simulink model "simulacionPID"  (R2020a)
settings: Solver=VariableStepAuto  StartTime=0.0  StopTime=10.0  RelTol=1e-3
undefined symbols (not defined in the file): x, xg, y, yg
settings Model: Creator=nacho  LastModifiedBy=nacho

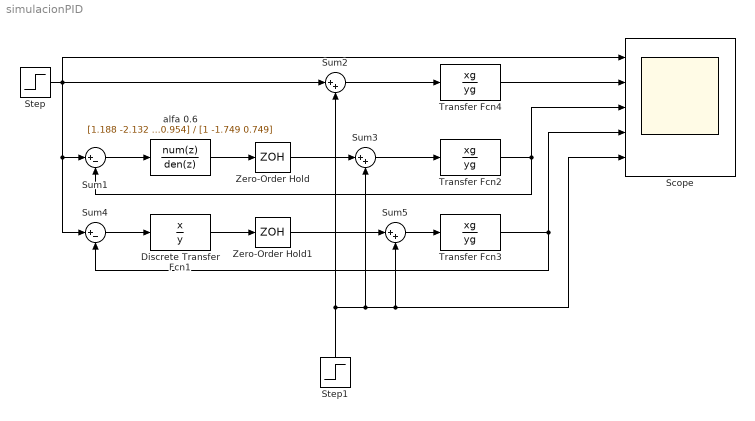
== system simulacionPID ==
  Discrete Transfer Fcn1 : DiscreteTransferFcn  Numerator=x  Denominator=y  SampleTime=0.03
  Scope : Scope  NumInputPorts=5
  Step : Step  Time=0.5  SampleTime=0.001
  Step1 : Step  Time=5  SampleTime=0.001
  Sum1 : Sum  Inputs=|+-
  Sum2 : Sum  Inputs=|++
  Sum3 : Sum  Inputs=|++
  Sum4 : Sum  Inputs=|+-
  Sum5 : Sum  Inputs=|++
  Transfer Fcn2 : TransferFcn  Numerator=xg  Denominator=yg
  Transfer Fcn3 : TransferFcn  Numerator=xg  Denominator=yg
  Transfer Fcn4 : TransferFcn  Numerator=xg  Denominator=yg
  Zero-Order Hold : ZeroOrderHold  SampleTime=0.03
  Zero-Order Hold1 : ZeroOrderHold  SampleTime=0.03
  alfa 0.6 : DiscreteTransferFcn  Numerator=[1.188 -2.132 0.954]  Denominator=[1 -1.749 0.749]  SampleTime=0.03
  wires:
  Transfer Fcn4/1 -> Scope/2
  Transfer Fcn2/1 -> Scope/3, Sum1/2
  alfa 0.6/1 -> Zero-Order Hold/1
  Sum1/1 -> alfa 0.6/1
  Sum2/1 -> Transfer Fcn4/1
  Zero-Order Hold/1 -> Sum3/1
  Sum3/1 -> Transfer Fcn2/1
  Discrete Transfer Fcn1/1 -> Zero-Order Hold1/1
  Step1/1 -> Scope/5, Sum5/2, Sum3/2, Sum2/2
  Transfer Fcn3/1 -> Scope/4, Sum4/2
  Step/1 -> Sum2/1, Scope/1, Sum4/1, Sum1/1
  Sum4/1 -> Discrete Transfer Fcn1/1
  Zero-Order Hold1/1 -> Sum5/1
  Sum5/1 -> Transfer Fcn3/1
